simulink model "DrawPlane"  (R2014b)
settings: Solver=ode45  StartTime=0.0  StopTime=10000  MaxStep=0.01  RelTol=1e-3
undefined symbols (not defined in the file or in its folder): drawplane
libraries: simulink x20
settings Model: Creator=CFRPG  LastModifiedBy=CFRPG

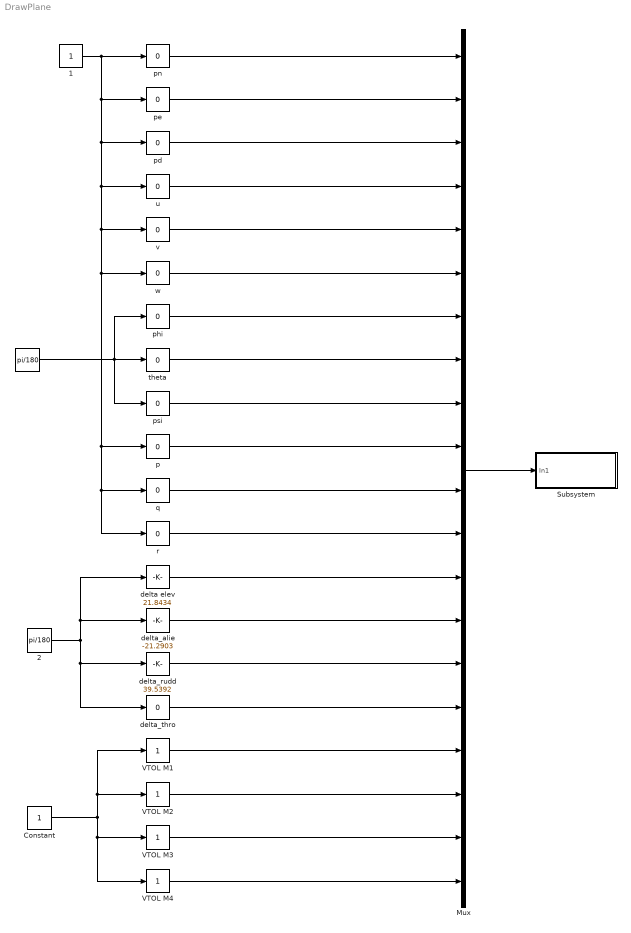
== system DrawPlane ==
  " " : Constant  Value=pi/180
  " 1" : Constant
  " 2" : Constant  Value=pi/180
  Constant : Constant
  Mux : Mux  Inputs=20
  Subsystem : Subsystem
  VTOL M{1..4} (4 alike) : simulink/Math Operations/Slider Gain  low=0  gain=1  high=2
  "delta elev " : simulink/Math Operations/Slider Gain  low=-60  gain=21.8434  high=60
  delta_alie : simulink/Math Operations/Slider Gain  low=-60  gain=-21.2903  high=60
  delta_rudd : simulink/Math Operations/Slider Gain  low=-60  gain=39.5392  high=60
  delta_thro : simulink/Math Operations/Slider Gain  low=-180  gain=0  high=180
  p : simulink/Math Operations/Slider Gain  low=-10  gain=0  high=10
  pd : simulink/Math Operations/Slider Gain  low=-10  gain=0  high=10
  pe : simulink/Math Operations/Slider Gain  low=-10  gain=0  high=10
  phi : simulink/Math Operations/Slider Gain  low=-180  gain=0  high=180
  "pn " : simulink/Math Operations/Slider Gain  low=-10  gain=0  high=10
  psi : simulink/Math Operations/Slider Gain  low=-180  gain=0  high=180
  q : simulink/Math Operations/Slider Gain  low=-10  gain=0  high=10
  r : simulink/Math Operations/Slider Gain  low=-10  gain=0  high=10
  theta : simulink/Math Operations/Slider Gain  low=-180  gain=0  high=180
  u : simulink/Math Operations/Slider Gain  low=-10  gain=0  high=10
  v : simulink/Math Operations/Slider Gain  low=-10  gain=0  high=10
  w : simulink/Math Operations/Slider Gain  low=-10  gain=0  high=10
  wires:
  " "/1 -> phi/1, theta/1, psi/1
  "pn "/1 -> Mux/1
  pe/1 -> Mux/2
  pd/1 -> Mux/3
  u/1 -> Mux/4
  v/1 -> Mux/5
  w/1 -> Mux/6
  phi/1 -> Mux/7
  theta/1 -> Mux/8
  psi/1 -> Mux/9
  p/1 -> Mux/10
  q/1 -> Mux/11
  r/1 -> Mux/12
  Mux/1 -> Subsystem/1(In1)
  " 1"/1 -> w/1, p/1, q/1, r/1, v/1, u/1, pd/1, pe/1, "pn "/1
  "delta elev "/1 -> Mux/13
  delta_alie/1 -> Mux/14
  delta_rudd/1 -> Mux/15
  " 2"/1 -> "delta elev "/1, delta_alie/1, delta_thro/1, delta_rudd/1
  delta_thro/1 -> Mux/16
  VTOL M1/1 -> Mux/17
  VTOL M2/1 -> Mux/18
  VTOL M3/1 -> Mux/19
  VTOL M4/1 -> Mux/20
  Constant/1 -> VTOL M2/1, VTOL M1/1, VTOL M3/1, VTOL M4/1

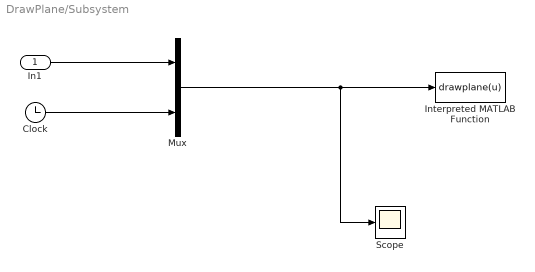
== system DrawPlane/Subsystem ==
  In1 : Inport
  Clock : Clock
  Interpreted MATLAB Function : MATLABFcn  MATLABFcn=drawplane(u)  OutputDimensions=0  Output1D=off
  Mux : Mux  Inputs=2
  Scope : Scope
  wires:
  In1/1 -> Mux/1
  Mux/1 -> Scope/1, Interpreted MATLAB Function/1
  Clock/1 -> Mux/2
